simulink model "blockdemo"  (Simulink 6.3)
settings: Solver=ode45  StartTime=0.0  StopTime=200  RelTol=1e-3
InitFcn:
  | %% DSPBuilder Start
  | alt_dspbuilder_update_model(bdroot)
  | %% DSPBuilder End
libraries: allblocks_alteradspbuilder2 x6
settings Model: Creator=cpurcell  LastModifiedBy=delphick
settings DebuggingCC: MultiTaskDSMMsg=error

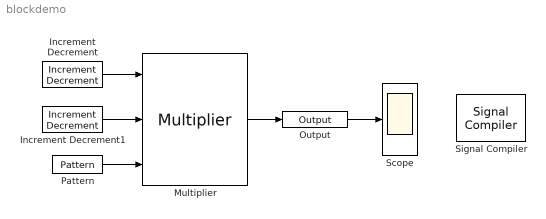
== system blockdemo ==
  Increment Decrement : allblocks_alteradspbuilder2/Increment Decrement  BusType=Signed Fractional  bwl=4  bwr=2  SpecifyClock=off  clr_value=0  direction=Increment  phase_selection=1  use_ena=off  use_sclr=off
  Increment Decrement1 : allblocks_alteradspbuilder2/Increment Decrement  BusType=Signed Fractional  bwl=2  bwr=4  SpecifyClock=off  clr_value=0  direction=Decrement  phase_selection=1  use_ena=off  use_sclr=off
  Multiplier : allblocks_alteradspbuilder2/Multiplier  BusType=Signed Fractional  bwl=4  bwr=2  pipeline=1  UseEqualInputWidth=off  bbwl=2  bbwr=4  FullResolution=off  OutputMsb=8  OutputLsb=0  OutputBwl=5  OutputBwr=4  UseDedicatedCircuitry=AUTO  use_ena=on  use_aclr=off
  Output : allblocks_alteradspbuilder2/Output  iofile=C:\workspace_clean\Documentation\DesignExamples\Tutorials\UnitBlocks\Arithmetic\Multiplier\tb_blockdemo\blockdemo_Output.capture  BusType=Inferred  bwl=8  bwr=0  PORTTYPE=Output
  Pattern : allblocks_alteradspbuilder2/Pattern  Sequence=1110110  SpecifyClock=off  use_ena=off  use_sclr=off
  Scope : Scope
      settings: TimeRange=200  YMin=-16.5  YMax=0.5
  Signal Compiler : allblocks_alteradspbuilder2/Signal Compiler  DeviceFamily=Stratix IV  DeviceName=AUTO  EnableSignalTap=off  SignalTapDepth=128  UseBoardBlock=off  StpUseDefaultClock=on  StpClock=clock
  wires:
  Increment Decrement/1 -> Multiplier/1
  Increment Decrement1/1 -> Multiplier/2
  Pattern/1 -> Multiplier/3
  Multiplier/1 -> Output/1
  Output/1 -> Scope/1
